simulink model "real_time_interface"  (R2022b)
settings: Solver=FixedStepDiscrete  StartTime=0  StopTime=inf  FixedStep=0.004  RelTol=1e-3  EnableMultiTasking=on
undefined symbols (not defined in the file or in its folder): UN
libraries: UnicornLib x1
settings Model: Creator=reitner  LastModifiedBy=William
settings SolverCC: AlgebraicLoopSolver=TrustRegion
settings DataIOCC: LimitDataPoints=on  SaveFormat=Array  ReturnWorkspaceOutputs=off
settings OptimizationCC: LifeSpan=inf
settings DebuggingCC: UnconnectedInputMsg=warning  UnconnectedOutputMsg=warning  UnconnectedLineMsg=warning  FrameProcessingCompatibilityMsg=none  SFUnexpectedBacktrackingDiag=warning  SFNoUnconditionalDefaultTransitionDiag=warning  SFExecutionAtInitializationDiag=none  SFMachineParentedDataDiag=warning  ArithmeticOperatorsInVariantConditions=warning
settings HardwareCC: ProdBitPerPointer=32  ProdBitPerSizeT=32  ProdBitPerPtrDiffT=32  ProdLargestAtomicFloat=None  ProdIntDivRoundTo=Undefined  ProdEndianess=Unspecified  ProdWordSize=32  ProdHWDeviceType=32-bit Generic
settings ModelReferenceCC: PropagateSignalLabelsOutOfModel=off
settings SFSimCC: SimUseLocalCustomCode=off  CustomCodeUndefinedFunction=UseInterfaceOnly
settings RTWCC: RTWUseLocalCustomCode=off
settings CodeAppCC: StateflowObjectComments=on
settings GRTTargetCC: TargetLangStandard=C89/C90 (ANSI)
settings ConfigComp: CovMetricSettings=dw  CovSaveCumulativeToWorkspaceVar=on  CovSaveSingleToWorkspaceVar=on  CovExternalEMLEnable=off

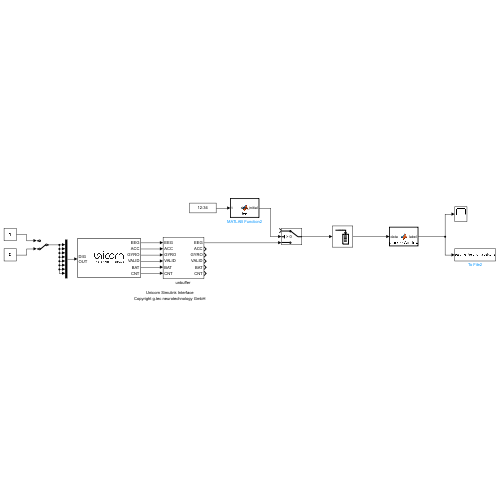
[thumbnail: Simulink's stored preview of the top-level diagram]
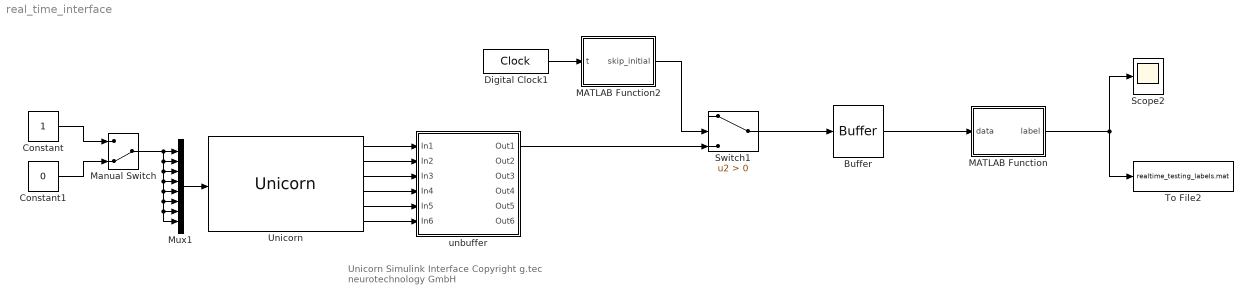
== system real_time_interface ==
  note: Unicorn Simulink Interface
      | Copyright g.tec neurotechnology GmbH
  Buffer : Buffer  N=250*5  OutputFrames=off
  Constant : Constant  OutDataTypeStr=boolean
  Constant1 : Constant  Value=0  OutDataTypeStr=boolean
  Digital Clock1 : DigitalClock  SampleTime=0.004
  MATLAB Function : MATLAB Function  TreatAsAtomicUnit=on
  MATLAB Function2 : MATLAB Function  TreatAsAtomicUnit=on
  Manual Switch : ManualSwitch  CurrentSetting=0
  Mux1 : Mux  Inputs=8
  Scope2 : Scope
  Switch1 : Switch  Criteria=u2 > Threshold  SaturateOnIntegerOverflow=off  InputSameDT=off
  To File2 : ToFile  Filename=realtime_testing_labels.mat  MatrixName=y
  Unicorn : UnicornLib/Unicorn  serial=UN-2019.02.58  old_serial=UN-2019.02.58  frame_length=1  input_source=Electrode
      settings: SourceProductName=Unicorn
  "unbuffer " : Subsystem
      mask Display:
      | port_label('input',1,'EEG')
      | port_label('input',2,'ACC')
      | port_label('input',3,'GYRO')
      | port_label('input',4,'VALID')
      | port_label('input',5,'BAT')
      | port_label('input',6,'CNT')
      | port_label('output',1,'EEG')
      | port_label('output',2,'ACC')
      | port_label('output',3,'GYRO')
      | port_label('output',4,'VALID')
      | port_label('output',5,'BAT')
      | port_label('output',6,'CNT')
  wires:
  "unbuffer "/1(Out1) -> Switch1/3
  Unicorn/1 -> "unbuffer "/1(In1)
  Unicorn/2 -> "unbuffer "/2(In2)
  Unicorn/3 -> "unbuffer "/3(In3)
  Unicorn/4 -> "unbuffer "/4(In4)
  Unicorn/5 -> "unbuffer "/5(In5)
  Unicorn/6 -> "unbuffer "/6(In6)
  Constant/1 -> Manual Switch/1
  Constant1/1 -> Manual Switch/2
  Mux1/1 -> Unicorn/1
  Manual Switch/1 -> Mux1/8, Mux1/7, Mux1/6, Mux1/5, Mux1/4, Mux1/3, Mux1/2, Mux1/1
  MATLAB Function/1(label) -> To File2/1, Scope2/1
  Digital Clock1/1 -> MATLAB Function2/1(t)
  MATLAB Function2/1(skip_initial) -> Switch1/2
  Switch1/1 -> Buffer/1
  Buffer/1 -> MATLAB Function/1(data)

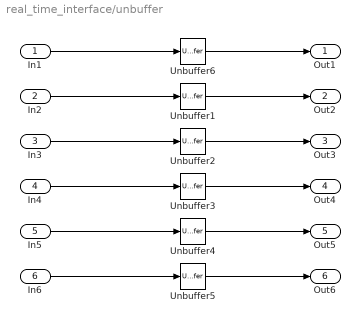
== system real_time_interface/unbuffer  ==
  In1 : Inport
  In2 : Inport  Port=2
  In3 : Inport  Port=3
  In4 : Inport  Port=4
  In5 : Inport  Port=5
  In6 : Inport  Port=6
  Unbuffer{1..6} (6 alike) : Unbuffer
  Out1 : Outport
  Out2 : Outport  Port=2
  Out3 : Outport  Port=3
  Out4 : Outport  Port=4
  Out5 : Outport  Port=5
  Out6 : Outport  Port=6
  wires:
  In1/1 -> Unbuffer6/1
  In6/1 -> Unbuffer5/1
  In2/1 -> Unbuffer1/1
  In3/1 -> Unbuffer2/1
  In4/1 -> Unbuffer3/1
  In5/1 -> Unbuffer4/1
  Unbuffer4/1 -> Out5/1
  Unbuffer5/1 -> Out6/1
  Unbuffer3/1 -> Out4/1
  Unbuffer2/1 -> Out3/1
  Unbuffer1/1 -> Out2/1
  Unbuffer6/1 -> Out1/1

== matlab function real_time_interface/MATLAB Function2 ==
  data: t input; skip_initial output
function skip_initial = fcn(t)
    skip_initial = 1;

    if t > 15
        skip_initial = 0;
    end
end

== matlab function real_time_interface/MATLAB Function ==
  data: data input; label output
function label = processWindow(data)
    coder.extrinsic('classify_epoch');
    
    % Initialize label to a default value
    label = 0;

    % Call the external script to classify the window
    label = classify_epoch(data);
end
